simulink model "ADCS_FunctionalArchitecture"  (R2024b)
settings: Solver=VariableStepAuto  StartTime=0.0  StopTime=10.0  RelTol=1e-3
settings Model: Creator=Ameya  LastModifiedBy=Ameya

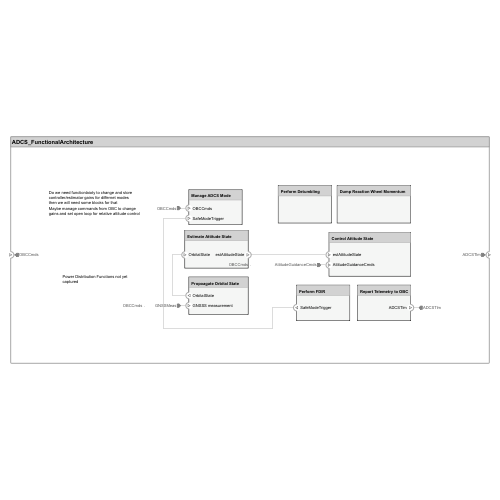
[thumbnail: Simulink's stored preview of the top-level diagram]
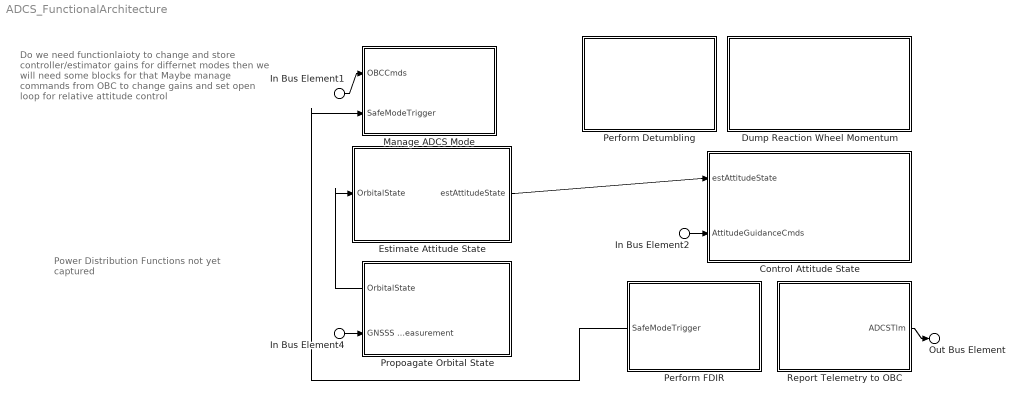
== system ADCS_FunctionalArchitecture ==
  note: Power Distribution Functions not yet
      | captured
  note: Do we need functionlaioty to change and store controller/estimator gains for differnet modes
      | then we will need some blocks for that
      | Maybe manage commands from OBC to change gains and set open loop for relative attitude control
  In Bus Element1 : Inport  PortName=OBCCmds
  In Bus Element2 : Inport  PortName=OBCCmds  Element=AttitudeGuidanceCmds
  In Bus Element4 : Inport  PortName=OBCCmds  Element=GNSSMeas
  Control Attitude State : Subsystem
      settings: PortSchema="{\"entries\":[{\"content\":{\"headerSize\":26,\"margin\":15,\"minimumSpacing\":25,\"sides\":[{\"content\":{\"connectorIds\":[\"In1\",\"In2\"]},\"type\":\"ConnectorPlacement.EquallySpacedRectSide\",\"uuid\":\"f9f0631b-ecc8-46b5-bc4b-a7110d617b31\"},{\"content\":{\"side\":\"RIGHT\"},\"type\":\"ConnectorPlacement.EquallySpacedRectSide\",\"uuid\":\"e25df8eb-9b9e-42fa-ad3a-7152061d4b64\"},{\"content\":{\"side\":\"TOP\"},\"type\":\"ConnectorPlacement.EquallySpacedRectSide\",\"uuid\":\"cf5f9ecc-bb1a-43e9-8f34-af7d7746aec9\"}]},\"type\":\"ConnectorPlacement.EquallySpacedConnector\",\"uuid\":\"cfe5eff4-6c86-4801-a4da-a0246b82223c\"}],\"packageUris\":[\"http://schema.mathworks.com/mf0/Connector/R2020b\"],\"version\":\"1.0\"}"
  Dump Reaction Wheel Momentum : Subsystem
      settings: PortSchema="{\"entries\":[{\"content\":{\"headerSize\":26,\"margin\":15,\"minimumSpacing\":25,\"sides\":[{\"content\":{},\"type\":\"ConnectorPlacement.EquallySpacedRectSide\",\"uuid\":\"f9f0631b-ecc8-46b5-bc4b-a7110d617b31\"},{\"content\":{\"side\":\"RIGHT\"},\"type\":\"ConnectorPlacement.EquallySpacedRectSide\",\"uuid\":\"e25df8eb-9b9e-42fa-ad3a-7152061d4b64\"},{\"content\":{\"side\":\"TOP\"},\"type\":\"ConnectorPlacement.EquallySpacedRectSide\",\"uuid\":\"cf5f9ecc-bb1a-43e9-8f34-af7d7746aec9\"}]},\"type\":\"ConnectorPlacement.EquallySpacedConnector\",\"uuid\":\"cfe5eff4-6c86-4801-a4da-a0246b82223c\"}],\"packageUris\":[\"http://schema.mathworks.com/mf0/Connector/R2020b\"],\"version\":\"1.0\"}"
  Estimate Attitude State : Subsystem
      settings: PortSchema="{\"entries\":[{\"content\":{\"headerSize\":26,\"margin\":15,\"minimumSpacing\":25,\"sides\":[{\"content\":{\"connectorIds\":[\"In1\"]},\"type\":\"ConnectorPlacement.EquallySpacedRectSide\",\"uuid\":\"f9f0631b-ecc8-46b5-bc4b-a7110d617b31\"},{\"content\":{\"connectorIds\":[\"Out1\"],\"side\":\"RIGHT\"},\"type\":\"ConnectorPlacement.EquallySpacedRectSide\",\"uuid\":\"e25df8eb-9b9e-42fa-ad3a-7152061d4b64\"},{\"content\":{\"side\":\"TOP\"},\"type\":\"ConnectorPlacement.EquallySpacedRectSide\",\"uuid\":\"cf5f9ecc-bb1a-43e9-8f34-af7d7746aec9\"},{\"content\":{\"side\":\"BOTTOM\"},\"type\":\"ConnectorPlacement.EquallySpacedRectSide\",\"uuid\":\"2a861a13-f865-4fc8-8906-f674af375b65\"}]},\"type\":\"ConnectorPlacement.EquallySpacedConnector\",\"uuid\":\"cfe5eff4-6c86-4801-a4da-a0246b82223c\"}],\"packageUris\":[\"http://schema.mathworks.com/mf0/Connector/R2020b\"],\"version\":\"1.0\"}"
  Manage ADCS Mode : Subsystem
      settings: PortSchema="{\"entries\":[{\"content\":{\"headerSize\":26,\"margin\":15,\"minimumSpacing\":25,\"sides\":[{\"content\":{\"connectorIds\":[\"In1\",\"In2\"]},\"type\":\"ConnectorPlacement.EquallySpacedRectSide\",\"uuid\":\"f9f0631b-ecc8-46b5-bc4b-a7110d617b31\"},{\"content\":{\"side\":\"RIGHT\"},\"type\":\"ConnectorPlacement.EquallySpacedRectSide\",\"uuid\":\"e25df8eb-9b9e-42fa-ad3a-7152061d4b64\"},{\"content\":{\"side\":\"TOP\"},\"type\":\"ConnectorPlacement.EquallySpacedRectSide\",\"uuid\":\"cf5f9ecc-bb1a-43e9-8f34-af7d7746aec9\"}]},\"type\":\"ConnectorPlacement.EquallySpacedConnector\",\"uuid\":\"cfe5eff4-6c86-4801-a4da-a0246b82223c\"}],\"packageUris\":[\"http://schema.mathworks.com/mf0/Connector/R2020b\"],\"version\":\"1.0\"}"
  Perform Detumbling : Subsystem
      settings: PortSchema="{\"entries\":[{\"content\":{\"headerSize\":26,\"margin\":15,\"minimumSpacing\":25,\"sides\":[{\"content\":{},\"type\":\"ConnectorPlacement.EquallySpacedRectSide\",\"uuid\":\"f9f0631b-ecc8-46b5-bc4b-a7110d617b31\"},{\"content\":{\"side\":\"RIGHT\"},\"type\":\"ConnectorPlacement.EquallySpacedRectSide\",\"uuid\":\"e25df8eb-9b9e-42fa-ad3a-7152061d4b64\"},{\"content\":{\"side\":\"TOP\"},\"type\":\"ConnectorPlacement.EquallySpacedRectSide\",\"uuid\":\"cf5f9ecc-bb1a-43e9-8f34-af7d7746aec9\"}]},\"type\":\"ConnectorPlacement.EquallySpacedConnector\",\"uuid\":\"cfe5eff4-6c86-4801-a4da-a0246b82223c\"}],\"packageUris\":[\"http://schema.mathworks.com/mf0/Connector/R2020b\"],\"version\":\"1.0\"}"
  Perform FDIR : Subsystem
      settings: PortSchema="{\"entries\":[{\"content\":{\"headerSize\":26,\"margin\":15,\"minimumSpacing\":25,\"sides\":[{\"content\":{\"connectorIds\":[\"Out1\"]},\"type\":\"ConnectorPlacement.EquallySpacedRectSide\",\"uuid\":\"f9f0631b-ecc8-46b5-bc4b-a7110d617b31\"},{\"content\":{\"side\":\"RIGHT\"},\"type\":\"ConnectorPlacement.EquallySpacedRectSide\",\"uuid\":\"e25df8eb-9b9e-42fa-ad3a-7152061d4b64\"},{\"content\":{\"side\":\"TOP\"},\"type\":\"ConnectorPlacement.EquallySpacedRectSide\",\"uuid\":\"cf5f9ecc-bb1a-43e9-8f34-af7d7746aec9\"}]},\"type\":\"ConnectorPlacement.EquallySpacedConnector\",\"uuid\":\"cfe5eff4-6c86-4801-a4da-a0246b82223c\"}],\"packageUris\":[\"http://schema.mathworks.com/mf0/Connector/R2020b\"],\"version\":\"1.0\"}"
  Propoagate Orbital State : Subsystem
      settings: PortSchema="{\"entries\":[{\"content\":{\"headerSize\":26,\"margin\":15,\"minimumSpacing\":25,\"sides\":[{\"content\":{\"connectorIds\":[\"Out1\",\"In1\"]},\"type\":\"ConnectorPlacement.EquallySpacedRectSide\",\"uuid\":\"f9f0631b-ecc8-46b5-bc4b-a7110d617b31\"},{\"content\":{\"side\":\"RIGHT\"},\"type\":\"ConnectorPlacement.EquallySpacedRectSide\",\"uuid\":\"e25df8eb-9b9e-42fa-ad3a-7152061d4b64\"},{\"content\":{\"side\":\"TOP\"},\"type\":\"ConnectorPlacement.EquallySpacedRectSide\",\"uuid\":\"cf5f9ecc-bb1a-43e9-8f34-af7d7746aec9\"}]},\"type\":\"ConnectorPlacement.EquallySpacedConnector\",\"uuid\":\"cfe5eff4-6c86-4801-a4da-a0246b82223c\"}],\"packageUris\":[\"http://schema.mathworks.com/mf0/Connector/R2020b\"],\"version\":\"1.0\"}"
  Report Telemetry to OBC : Subsystem
      settings: PortSchema="{\"entries\":[{\"content\":{\"headerSize\":26,\"margin\":15,\"minimumSpacing\":25,\"sides\":[{\"content\":{},\"type\":\"ConnectorPlacement.EquallySpacedRectSide\",\"uuid\":\"f9f0631b-ecc8-46b5-bc4b-a7110d617b31\"},{\"content\":{\"connectorIds\":[\"Out1\"],\"side\":\"RIGHT\"},\"type\":\"ConnectorPlacement.EquallySpacedRectSide\",\"uuid\":\"e25df8eb-9b9e-42fa-ad3a-7152061d4b64\"},{\"content\":{\"side\":\"TOP\"},\"type\":\"ConnectorPlacement.EquallySpacedRectSide\",\"uuid\":\"cf5f9ecc-bb1a-43e9-8f34-af7d7746aec9\"}]},\"type\":\"ConnectorPlacement.EquallySpacedConnector\",\"uuid\":\"cfe5eff4-6c86-4801-a4da-a0246b82223c\"}],\"packageUris\":[\"http://schema.mathworks.com/mf0/Connector/R2020b\"],\"version\":\"1.0\"}"
  Out Bus Element : Outport  PortName=ADCSTlm
  wires:
  Report Telemetry to OBC/1(ADCSTlm) -> Out Bus Element/1
  In Bus Element1/1 -> Manage ADCS Mode/1(OBCCmds)
  Estimate Attitude State/1(estAttitudeState) -> Control Attitude State/1(estAttitudeState)
  Perform FDIR/1(SafeModeTrigger) -> Manage ADCS Mode/2(SafeModeTrigger)
  In Bus Element2/1 -> Control Attitude State/2(AttitudeGuidanceCmds)
  Propoagate Orbital State/1(OrbitalState) -> Estimate Attitude State/1(OrbitalState)
  In Bus Element4/1 -> Propoagate Orbital State/1(GNSSS measurement)

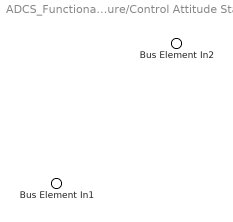
== system ADCS_FunctionalArchitecture/Control Attitude State ==
  Bus Element In2 : Inport  PortName=estAttitudeState
  Bus Element In1 : Inport  Port=2  PortName=AttitudeGuidanceCmds

== system ADCS_FunctionalArchitecture/Dump Reaction Wheel Momentum ==

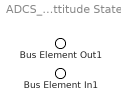
== system ADCS_FunctionalArchitecture/Estimate Attitude State ==
  Bus Element In1 : Inport  PortName=OrbitalState
  Bus Element Out1 : Outport  PortName=estAttitudeState

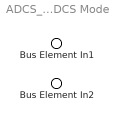
== system ADCS_FunctionalArchitecture/Manage ADCS Mode ==
  Bus Element In1 : Inport  PortName=OBCCmds
  Bus Element In2 : Inport  Port=2  PortName=SafeModeTrigger

== system ADCS_FunctionalArchitecture/Perform Detumbling ==

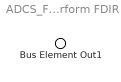
== system ADCS_FunctionalArchitecture/Perform FDIR ==
  Bus Element Out1 : Outport  PortName=SafeModeTrigger

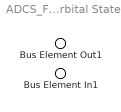
== system ADCS_FunctionalArchitecture/Propoagate Orbital State ==
  Bus Element In1 : Inport  PortName=GNSSS measurement
  Bus Element Out1 : Outport  PortName=OrbitalState

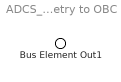
== system ADCS_FunctionalArchitecture/Report Telemetry to OBC ==
  Bus Element Out1 : Outport  PortName=ADCSTlm
